simulink model "second"  (R2023a)
settings: Solver=VariableStepAuto  StartTime=0.0  StopTime=10  FixedStep=0.01  RelTol=1e-3
settings Model: Creator=evdokiiagalkina  LastModifiedBy=evdokiiagalkina

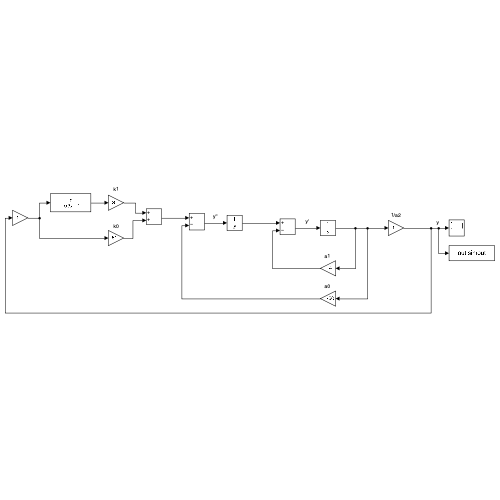
[thumbnail: Simulink's stored preview of the top-level diagram]
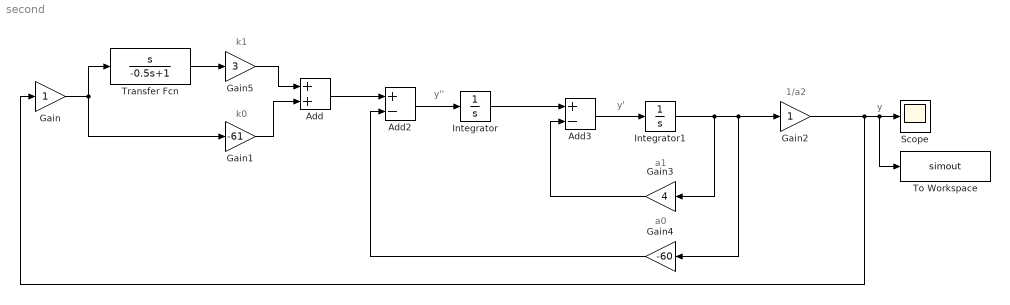
== system second ==
  note: k1
  note: a1
  note: y''
  note: k0
  note: a0
  note: 1/a2
  note: y'
  note: y
  Add : Sum
  Add2 : Sum  Inputs=+-
  Add3 : Sum  Inputs=+-
  Gain : Gain
  Gain1 : Gain  Gain=-61
  Gain2 : Gain
  Gain3 : Gain  Gain=4
  Gain4 : Gain  Gain=-60
  Gain5 : Gain  Gain=3
  Integrator : Integrator  InitialCondition=5
  Integrator1 : Integrator  InitialCondition=5
  Scope : Scope
  To Workspace : ToWorkspace  VariableName=simout  SaveFormat=Timeseries  SampleTime=-1
  Transfer Fcn : TransferFcn  Numerator=[1 0]  Denominator=[-0.5 1]
  wires:
  Add2/1 -> Integrator/1
  Integrator/1 -> Add3/1
  Gain2/1 -> Gain/1, To Workspace/1, Scope/1
  Gain/1 -> Transfer Fcn/1, Gain1/1
  Add3/1 -> Integrator1/1
  Gain1/1 -> Add/2
  Add/1 -> Add2/1
  Gain3/1 -> Add3/2
  Integrator1/1 -> Gain3/1, Gain4/1, Gain2/1
  Gain4/1 -> Add2/2
  Transfer Fcn/1 -> Gain5/1
  Gain5/1 -> Add/1
